simulink model "velocityContinuousControl"  (R2017a)
settings: Solver=VariableStepAuto  StartTime=0.0  StopTime=10.0  RelTol=1e-3
values from neighbouring files (symbols this model uses):
  dm = 2.96e-5    (= 2.96e-05)    [parameter.m]
  J = 2.37e-5    (= 2.37e-05)    [parameter.m]
  Ke = 1 / sc * 60 / 2 / pi    (= 0.0697028947848)    [parameter.m]
  Ki = c*c*(Ke*Kt+R*dm+P*Kt)^2 / Kt/J/R    [continuousVelocityPControl.m]
  Kp = (2*c-1)*(Ke*Kt+R*dm)/Kt + 2*c*P    [continuousVelocityPControl.m]    (also in parameter.m = 0.1)
  Kt = 69.7e-3    (= 0.0697)    [parameter.m]
  L = 11.4e-3    (= 0.0114)    [parameter.m]
  P = 0.1    [continuousVelocityPControl.m]
  P_design = -c*(Ke*Kt+R*dm+P*Kt)/J/R    [continuousVelocityPControl.m]
  R = 112    [parameter.m]
  t0 = J*R*(Kt*Ke+R*dm+Kt*Ki)/(Kt*c*(Ke*Kt+R*dm+P*Kt))    [continuousVelocityPControl.m]
  Tc = 1e-3    (= 0.001)    [parameter.m]
settings Model: Creator=99641  LastModifiedBy=99641

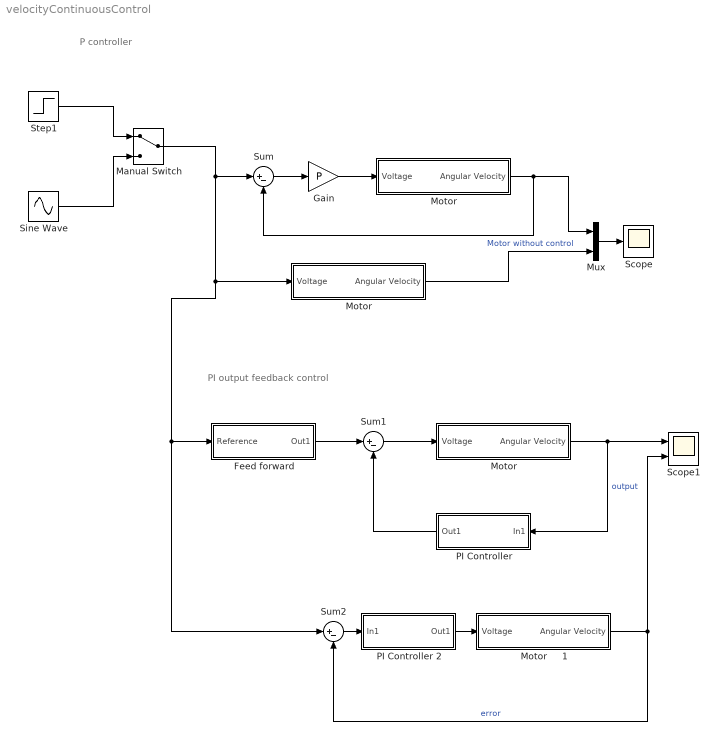
== system velocityContinuousControl ==
  note: PI output feedback control
  note: P controller
  "Feed forward " : Subsystem
  Gain : Gain  Gain=P
  Manual Switch : ManualSwitch
  Motor : Subsystem
  "Motor " : Subsystem
  "Motor     " : Subsystem
  Motor     1 : Subsystem
  Mux : Mux  Inputs=2
  "PI Controller " : Subsystem
  PI Controller 2 : Subsystem
  Scope : Scope
  Scope1 : Scope  NumInputPorts=2
  Sine Wave : Sin  Amplitude=20  SampleTime=0
  Step1 : Step  After=20  SampleTime=0
  Sum : Sum  Inputs=|+-
  Sum1 : Sum  Inputs=|+-
  Sum2 : Sum  Inputs=|+-
  wires:
  Step1/1 -> Manual Switch/1
  Gain/1 -> "Motor "/1(Voltage)
  Sum/1 -> Gain/1
  Motor/1(Angular Velocity) -> Mux/2  "Motor without control"
  Mux/1 -> Scope/1
  "Motor "/1(Angular Velocity) -> Sum/2, Mux/1
  Sine Wave/1 -> Manual Switch/2
  "PI Controller "/1(Out1) -> Sum1/2
  "Feed forward "/1(Out1) -> Sum1/1
  Sum1/1 -> "Motor     "/1(Voltage)
  "Motor     "/1(Angular Velocity) -> "PI Controller "/1(In1), Scope1/1  "output"
  Sum2/1 -> PI Controller 2/1(In1)
  Manual Switch/1 -> Sum2/1, "Feed forward "/1(Reference), Motor/1(Voltage), Sum/1
  Motor     1/1(Angular Velocity) -> Scope1/2, Sum2/2  "error"
  PI Controller 2/1(Out1) -> Motor     1/1(Voltage)

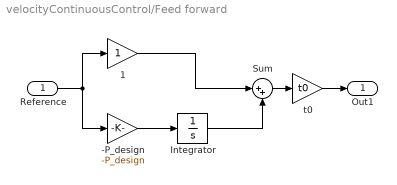
== system velocityContinuousControl/Feed forward  ==
  Reference : Inport
  "-P_design " : Gain  Gain=-P_design
  "1 " : Gain
  Integrator : Integrator
  Sum : Sum  Inputs=|++
  t0 : Gain  Gain=t0
  Out1 : Outport
  wires:
  Reference/1 -> "-P_design "/1, "1 "/1
  "1 "/1 -> Sum/1
  Integrator/1 -> Sum/2
  "-P_design "/1 -> Integrator/1
  Sum/1 -> t0/1
  t0/1 -> Out1/1

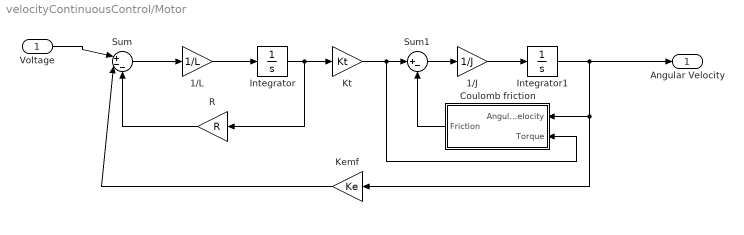
== system velocityContinuousControl/Motor ==
  Voltage : Inport
  1/J : Gain  Gain=1/J
  1/L : Gain  Gain=1/L
  Coulomb friction : Subsystem
  Integrator : Integrator
  Integrator1 : Integrator
  Kemf : Gain  Gain=Ke
  "Kt " : Gain  Gain=Kt
  R : Gain  Gain=R
  Sum : Sum  Inputs=|+--
  Sum1 : Sum  Inputs=|+-
  Angular Velocity : Outport
  wires:
  Coulomb friction/1("Friction ") -> Sum1/2
  Kemf/1 -> Sum/2
  Integrator/1 -> "Kt "/1, R/1
  1/L/1 -> Integrator/1
  Integrator1/1 -> Coulomb friction/1(Angular Velocity), Kemf/1, Angular Velocity/1
  Sum1/1 -> 1/J/1
  "Kt "/1 -> Sum1/1, Coulomb friction/2("Torque ")
  1/J/1 -> Integrator1/1
  R/1 -> Sum/3
  Voltage/1 -> Sum/1
  Sum/1 -> 1/L/1

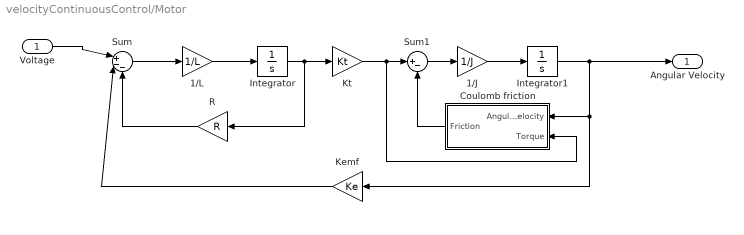
== system velocityContinuousControl/Motor  ==
  Voltage : Inport
  1/J : Gain  Gain=1/J
  1/L : Gain  Gain=1/L
  Coulomb friction : Subsystem
  Integrator : Integrator
  Integrator1 : Integrator
  Kemf : Gain  Gain=Ke
  "Kt " : Gain  Gain=Kt
  R : Gain  Gain=R
  Sum : Sum  Inputs=|+--
  Sum1 : Sum  Inputs=|+-
  Angular Velocity : Outport
  wires:
  Sum/1 -> 1/L/1
  Voltage/1 -> Sum/1
  R/1 -> Sum/3
  1/J/1 -> Integrator1/1
  "Kt "/1 -> Coulomb friction/2("Torque "), Sum1/1
  Sum1/1 -> 1/J/1
  Integrator1/1 -> Angular Velocity/1, Kemf/1, Coulomb friction/1(Angular Velocity)
  1/L/1 -> Integrator/1
  Integrator/1 -> R/1, "Kt "/1
  Kemf/1 -> Sum/2
  Coulomb friction/1("Friction ") -> Sum1/2

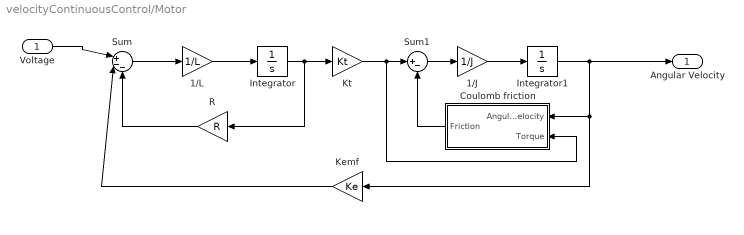
== system velocityContinuousControl/Motor      ==
  Voltage : Inport
  1/J : Gain  Gain=1/J
  1/L : Gain  Gain=1/L
  Coulomb friction : Subsystem
  Integrator : Integrator
  Integrator1 : Integrator
  Kemf : Gain  Gain=Ke
  "Kt " : Gain  Gain=Kt
  R : Gain  Gain=R
  Sum : Sum  Inputs=|+--
  Sum1 : Sum  Inputs=|+-
  Angular Velocity : Outport
  wires:
  Sum/1 -> 1/L/1
  Voltage/1 -> Sum/1
  R/1 -> Sum/3
  1/J/1 -> Integrator1/1
  "Kt "/1 -> Coulomb friction/2("Torque "), Sum1/1
  Sum1/1 -> 1/J/1
  Integrator1/1 -> Angular Velocity/1, Kemf/1, Coulomb friction/1(Angular Velocity)
  1/L/1 -> Integrator/1
  Integrator/1 -> R/1, "Kt "/1
  Kemf/1 -> Sum/2
  Coulomb friction/1("Friction ") -> Sum1/2

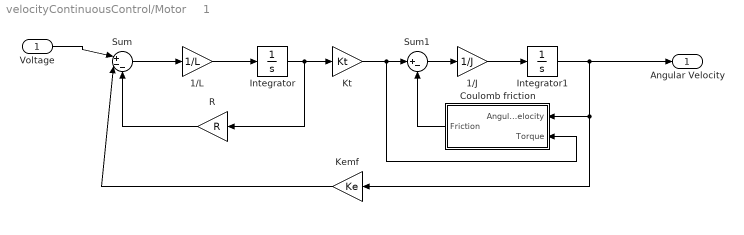
== system velocityContinuousControl/Motor     1 ==
  Voltage : Inport
  1/J : Gain  Gain=1/J
  1/L : Gain  Gain=1/L
  Coulomb friction : Subsystem
  Integrator : Integrator
  Integrator1 : Integrator
  Kemf : Gain  Gain=Ke
  "Kt " : Gain  Gain=Kt
  R : Gain  Gain=R
  Sum : Sum  Inputs=|+--
  Sum1 : Sum  Inputs=|+-
  Angular Velocity : Outport
  wires:
  Coulomb friction/1("Friction ") -> Sum1/2
  Kemf/1 -> Sum/2
  Integrator/1 -> "Kt "/1, R/1
  1/L/1 -> Integrator/1
  Integrator1/1 -> Coulomb friction/1(Angular Velocity), Kemf/1, Angular Velocity/1
  Sum1/1 -> 1/J/1
  "Kt "/1 -> Sum1/1, Coulomb friction/2("Torque ")
  1/J/1 -> Integrator1/1
  R/1 -> Sum/3
  Voltage/1 -> Sum/1
  Sum/1 -> 1/L/1

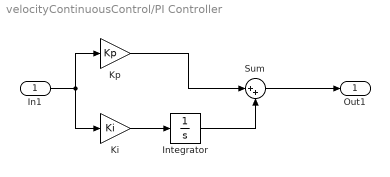
== system velocityContinuousControl/PI Controller  ==
  In1 : Inport
  Integrator : Integrator
  "Ki " : Gain  Gain=Ki
  Kp : Gain  Gain=Kp
  Sum : Sum  Inputs=|++
  Out1 : Outport
  wires:
  Sum/1 -> Out1/1
  "Ki "/1 -> Integrator/1
  Integrator/1 -> Sum/2
  Kp/1 -> Sum/1
  In1/1 -> Kp/1, "Ki "/1

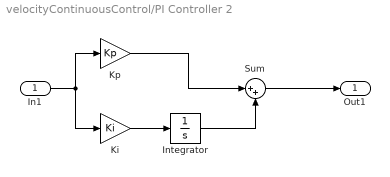
== system velocityContinuousControl/PI Controller 2 ==
  In1 : Inport
  Integrator : Integrator
  "Ki " : Gain  Gain=Ki
  Kp : Gain  Gain=Kp
  Sum : Sum  Inputs=|++
  Out1 : Outport
  wires:
  Sum/1 -> Out1/1
  "Ki "/1 -> Integrator/1
  Integrator/1 -> Sum/2
  Kp/1 -> Sum/1
  In1/1 -> Kp/1, "Ki "/1

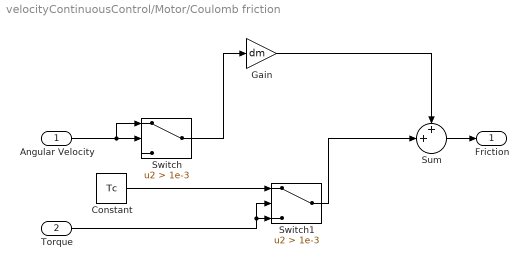
== system velocityContinuousControl/Motor/Coulomb friction ==
  Angular Velocity : Inport
  "Torque " : Inport  Port=2
  Constant : Constant  Value=Tc
  Gain : Gain  Gain=dm
  Sum : Sum  Inputs=++|
  Switch : Switch  Criteria=u2 > Threshold  Threshold=1e-3
  Switch1 : Switch  Criteria=u2 > Threshold  Threshold=1e-3
  "Friction " : Outport
  wires:
  Constant/1 -> Switch1/1
  "Torque "/1 -> Switch1/2, Switch1/3
  Switch/1 -> Gain/1
  Angular Velocity/1 -> Switch/2, Switch/1
  Sum/1 -> "Friction "/1
  Gain/1 -> Sum/1
  Switch1/1 -> Sum/2

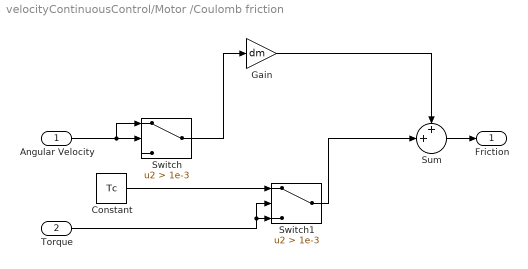
== system velocityContinuousControl/Motor /Coulomb friction ==
  Angular Velocity : Inport
  "Torque " : Inport  Port=2
  Constant : Constant  Value=Tc
  Gain : Gain  Gain=dm
  Sum : Sum  Inputs=++|
  Switch : Switch  Criteria=u2 > Threshold  Threshold=1e-3
  Switch1 : Switch  Criteria=u2 > Threshold  Threshold=1e-3
  "Friction " : Outport
  wires:
  Switch1/1 -> Sum/2
  Gain/1 -> Sum/1
  Sum/1 -> "Friction "/1
  Angular Velocity/1 -> Switch/1, Switch/2
  Switch/1 -> Gain/1
  "Torque "/1 -> Switch1/3, Switch1/2
  Constant/1 -> Switch1/1

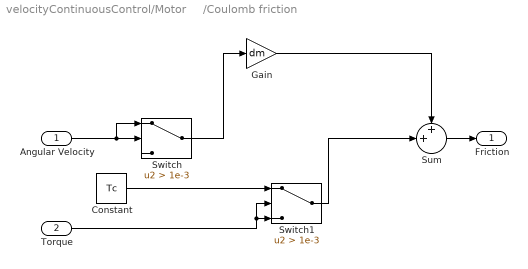
== system velocityContinuousControl/Motor     /Coulomb friction ==
  Angular Velocity : Inport
  "Torque " : Inport  Port=2
  Constant : Constant  Value=Tc
  Gain : Gain  Gain=dm
  Sum : Sum  Inputs=++|
  Switch : Switch  Criteria=u2 > Threshold  Threshold=1e-3
  Switch1 : Switch  Criteria=u2 > Threshold  Threshold=1e-3
  "Friction " : Outport
  wires:
  Switch1/1 -> Sum/2
  Gain/1 -> Sum/1
  Sum/1 -> "Friction "/1
  Angular Velocity/1 -> Switch/1, Switch/2
  Switch/1 -> Gain/1
  "Torque "/1 -> Switch1/3, Switch1/2
  Constant/1 -> Switch1/1

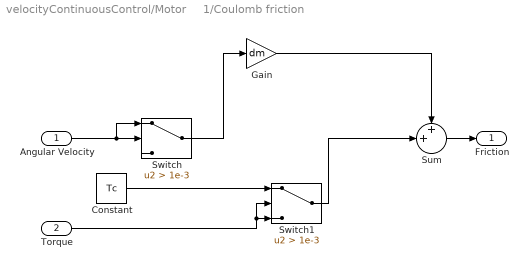
== system velocityContinuousControl/Motor     1/Coulomb friction ==
  Angular Velocity : Inport
  "Torque " : Inport  Port=2
  Constant : Constant  Value=Tc
  Gain : Gain  Gain=dm
  Sum : Sum  Inputs=++|
  Switch : Switch  Criteria=u2 > Threshold  Threshold=1e-3
  Switch1 : Switch  Criteria=u2 > Threshold  Threshold=1e-3
  "Friction " : Outport
  wires:
  Constant/1 -> Switch1/1
  "Torque "/1 -> Switch1/2, Switch1/3
  Switch/1 -> Gain/1
  Angular Velocity/1 -> Switch/2, Switch/1
  Sum/1 -> "Friction "/1
  Gain/1 -> Sum/1
  Switch1/1 -> Sum/2
